simulink model "FloatingPointSystem"  (R2021b)
settings: Solver=FixedStepDiscrete  StartTime=0.0  StopTime=0.0001  FixedStep=1/312.5e6  RelTol=1e-3
model workspace (MAT data in the model file):
  test = 0
libraries: dsphdlxfrm x3, simulink x1, hdlsllib x1
settings Model: DataTypeOverride=Off  FPTShortcutValueString='{{},{''BaselineRun'',1,1,1,''BaselineRun'','''',{},''M'',''F'',''''},{''EmbeddedRun'',1,1,1,''EmbeddedRun'','''',{},''M'','''',''''}}'  Creator=max_d  LastModifiedBy=max_d
settings SolverCC: AlgebraicLoopSolver=TrustRegion  AutoInsertRateTranBlk=on
settings DataIOCC: LimitDataPoints=on  SaveOutput=off  SaveTime=off
settings OptimizationCC: BlockReduction=off  ConditionallyExecuteInputs=off  DefaultParameterBehavior=Inlined  InheritOutputTypeSmallerThanSingle=on  LifeSpan=inf
settings DebuggingCC: SignalRangeChecking=warning  AlgebraicLoopMsg=error  SingleTaskRateTransMsg=error  AllowSymbolicDim=off  StrictBusMsg=ErrorOnBusTreatedAsVector  SFUnexpectedBacktrackingDiag=warning  SFNoUnconditionalDefaultTransitionDiag=warning  SFExecutionAtInitializationDiag=none  SFMachineParentedDataDiag=warning  ArithmeticOperatorsInVariantConditions=warning
settings HardwareCC: ProdBitPerPointer=32  ProdBitPerSizeT=32  ProdBitPerPtrDiffT=32  ProdLargestAtomicFloat=None  ProdIntDivRoundTo=Undefined  ProdEndianess=Unspecified  ProdWordSize=32  ProdHWDeviceType=ASIC/FPGA->ASIC/FPGA  ProdEqTarget=off
settings SFSimCC: SimUseLocalCustomCode=off  CustomCodeUndefinedFunction=UseInterfaceOnly
settings RTWCC: RTWUseLocalCustomCode=off
settings CodeAppCC: StateflowObjectComments=on
settings GRTTargetCC: TargetLangStandard=C89/C90 (ANSI)
settings ConfigComp: CovScope=ReferencedModels  CovMetricSettings=dw  CovSaveCumulativeToWorkspaceVar=on  CovSaveSingleToWorkspaceVar=on  CovExternalEMLEnable=off  CovSFcnEnable=off

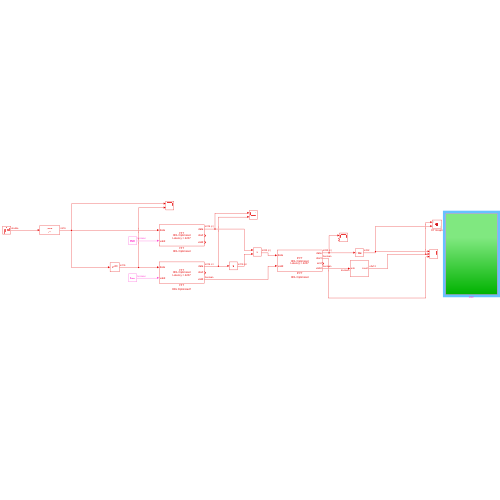
[thumbnail: Simulink's stored preview of the top-level diagram]
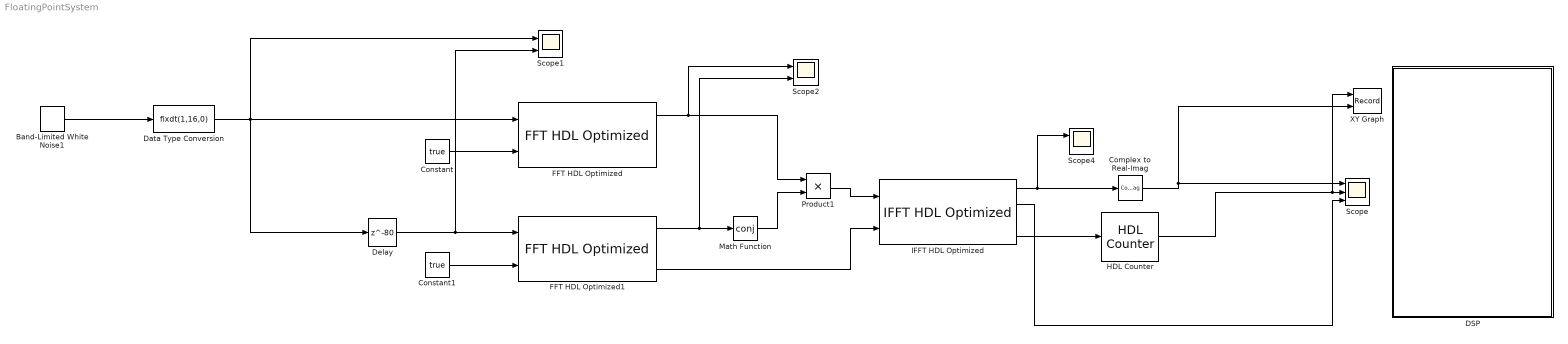
== system FloatingPointSystem ==
  Band-Limited White Noise1 : simulink/Sources/Band-Limited White Noise  Cov=[0.1]  Ts=1/312.5e6  seed=[23341]
  Complex to Real-Imag : ComplexToRealImag  Output=Real
  Constant : Constant  Value=true
  Constant1 : Constant  Value=true
  DSP : Subsystem
  Data Type Conversion : DataTypeConversion  OutDataTypeStr=fixdt(1,16,0)  ConvertRealWorld=Stored Integer (SI)
  Delay : Delay  DelayLength=80  InitialCondition=0
  FFT HDL Optimized : dsphdlxfrm/FFT HDL Optimized  FFTLength=4096  Architecture=Streaming Radix 2^2  ComplexMultiplication=Use 4 multipliers and 2 adders  BitReversedOutput=on  BitReversedInput=off  Normalize=on  SimulateUsing=Code generation  RoundingMethod=Floor  ResetInputPort=off  StartOutputPort=on  EndOutputPort=off
      settings: SourceProductBaseCode=DS
  FFT HDL Optimized1 : dsphdlxfrm/FFT HDL Optimized  FFTLength=4096  Architecture=Streaming Radix 2^2  ComplexMultiplication=Use 4 multipliers and 2 adders  BitReversedOutput=on  BitReversedInput=off  Normalize=on  SimulateUsing=Code generation  RoundingMethod=Floor  ResetInputPort=off  StartOutputPort=on  EndOutputPort=off
      settings: SourceProductBaseCode=DS
  HDL Counter : hdlsllib/Sources/HDL Counter  CountType=Count limited  CountInit=4095  CountStep=-1  CountMax=0  CountFromType=Initial value  CountFrom=4095  CountResetPort=off  CountLoadPort=off  CountEnbPort=on  CountDirPort=off  CountHitOutputPort=off  CountDataType=Unsigned  CountWordLen=12  CountFracLen=0  CountSampTime=1
  IFFT HDL Optimized : dsphdlxfrm/IFFT HDL Optimized  FFTLength=4096  Architecture=Streaming Radix 2^2  ComplexMultiplication=Use 4 multipliers and 2 adders  BitReversedOutput=off  BitReversedInput=on  Normalize=on  SimulateUsing=Code generation  RoundingMethod=Floor  ResetInputPort=off  StartOutputPort=on  EndOutputPort=on
      settings: SourceProductBaseCode=DS
  Math Function : Math  Operator=conj  SaturateOnIntegerOverflow=on
  Product1 : Product
  Scope : Scope  NumInputPorts=3
  Scope1 : Scope  NumInputPorts=2
  Scope2 : Scope  NumInputPorts=2
  Scope4 : Scope  NumInputPorts=2
  XY Graph : Record  FileSettingsInternal="{\"entries\":[{\"content\":{\"excelSettings\":{\"content\":{},\"type\":\"Streamout.ExcelSettings\"}},\"type\":\"Streamout.FileSettingStorage\",\"uuid\":\"b44be613-558b-472d-8dec-aa5bded21848\"}],\"packageUris\":[\"http://schema.mathworks.com/mf0/streamout_blocks/R2020a\"],\"version\":\"1.0\"}"  Layout=[1 1]  SignalsInternal="{\"entries\":[{\"content\":{\"signals\":[{\"content\":{\"blockPath\":[\"System_Template/XY Graph\"],\"channel\":[],\"dimensions\":[1],\"domain\":\"System_Template/XY Graph\",\"lineColor\":\"#a2142f\",\"plots\":[1],\"port\":1,\"sid\":[\"\"],\"signalID\":860,\"signalName\":\"HDL Counter\"},\"type\":\"RecordBlkView.Signal\",\"uuid\":\"a7cc4d68-4c8c-4b30-902e-c34036ab9f0b\"},{\"content\":{\"blockPath\":[\"System_Template/XY Graph\"],\"channel\":[],\"dimensions\":[1,1],\"domain\":\"System_Template/XY Graph\",\"lineColor\":\"#139fff\",\"plots\":[1],\"port\":2,\"sid\":[\"\"],\"signalID\":864,\"signalName\":\"Complex to\\nReal-Imag\"},\"type\":\"RecordBlkView.Signal\",\"uuid\":\"97637e3b-5635-443c-872a-8a950910aeef\"}]},\"type\":\"RecordBlkView.InputSignals\",\"uuid\":\"1dd11390-d5af-4420-97e8-227899983e51\"}],\"packageUris\":[\"http://schema.mathworks.com/mf0/streamout_blocks/R2020a\"],\"version\":\"1.0\"}"  VisualizationBindings="{\"xyplotplugin\":{\"info\":[{\"series\":[{\"bindingParametersList\":[{\"parameter\":\"X-Axis\",\"signalID\":860,\"signalName\":\"HDL Counter\"},{\"parameter\":\"Y-Axis\",\"signalID\":864,\"signalName\":\"Complex to\\nReal-Imag\"}],\"seriesID\":49152}],\"subplotID\":1}]}}"  CompatibilityTag=XY
  wires:
  Constant/1 -> FFT HDL Optimized/2
  Delay/1 -> Scope1/2, FFT HDL Optimized1/1
  Constant1/1 -> FFT HDL Optimized1/2
  FFT HDL Optimized1/1 -> Scope2/2, Math Function/1
  FFT HDL Optimized/1 -> Scope2/1, Product1/1
  Math Function/1 -> Product1/2
  Product1/1 -> IFFT HDL Optimized/1
  IFFT HDL Optimized/1 -> Scope4/1, Complex to Real-Imag/1
  FFT HDL Optimized1/3 -> IFFT HDL Optimized/2
  Band-Limited White Noise1/1 -> Data Type Conversion/1
  IFFT HDL Optimized/2 -> Scope/3
  Data Type Conversion/1 -> Scope1/1, Delay/1, FFT HDL Optimized/1
  Complex to Real-Imag/1 -> XY Graph/2, Scope/1
  IFFT HDL Optimized/4 -> HDL Counter/1
  HDL Counter/1 -> XY Graph/1, Scope/2

== system FloatingPointSystem/DSP ==
